simulink model "Trabalho8_2A_Simulink"  (R2022b)
settings: Solver=VariableStepAuto  StartTime=0.0  StopTime=10.0  RelTol=1e-3
undefined symbols (not defined in the file or in its folder): B, C, g, I, L, M, m
settings Model: Creator=brunofavs  LastModifiedBy=brunofavs

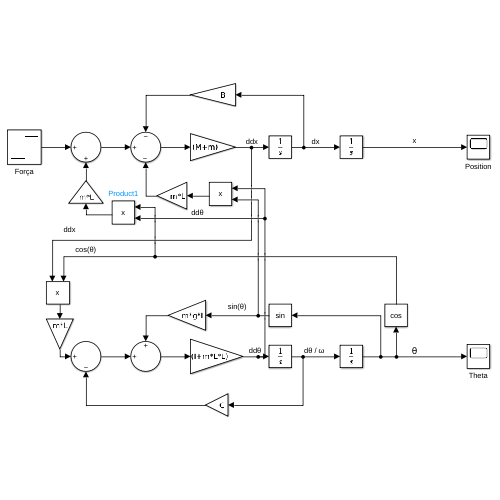
[thumbnail: Simulink's stored preview of the top-level diagram]
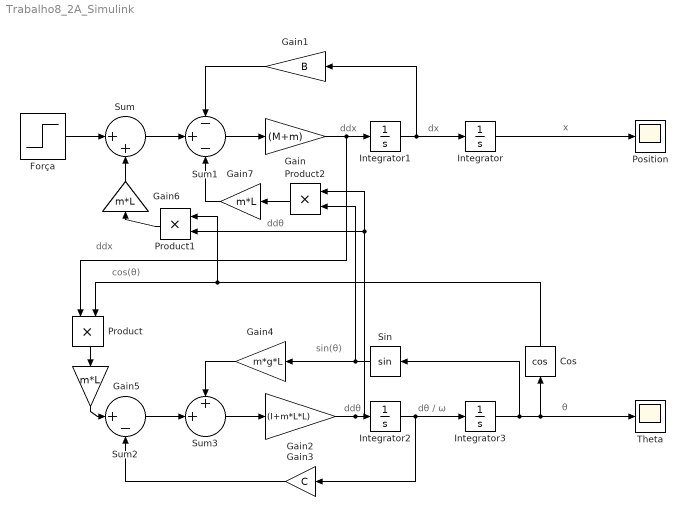
== system Trabalho8_2A_Simulink ==
  note: cos(θ)
  note: sin(θ)
  note: dθ / ω
  note: θ
  note: ddx
  note: dx
  note: x
  note: ddθ
  note: ddx
  note: ddθ
  Cos : Trigonometry  Operator=cos
  Força : Step  After=0.5  SampleTime=0
  Gain : Gain  Gain=(M+m)
  Gain1 : Gain  Gain=B
  Gain2 : Gain  Gain=(I+m*L*L)
  Gain3 : Gain  Gain=C
  Gain4 : Gain  Gain=m*g*L
  Gain5 : Gain  Gain=m*L
  Gain6 : Gain  Gain=m*L
  Gain7 : Gain  Gain=m*L
  Integrator{,1..3} (4 alike) : Integrator
  Position : Scope
  Product : Product
  Product1 : Product
  Product2 : Product
  Sin : Trigonometry
  Sum : Sum  Inputs=|++
  Sum1 : Sum  Inputs=-+-
  Sum2 : Sum  Inputs=|+-
  Sum3 : Sum  Inputs=++|
  Theta : Scope
  wires:
  Integrator1/1 -> Gain1/1, Integrator/1
  Integrator/1 -> Position/1
  Integrator2/1 -> Gain3/1, Integrator3/1
  Integrator3/1 -> Cos/1, Theta/1, Sin/1
  Sum/1 -> Sum1/2
  Força/1 -> Sum/1
  Gain/1 -> Product/1, Integrator1/1
  Sum1/1 -> Gain/1
  Gain1/1 -> Sum1/1
  Gain2/1 -> Product2/1, Product1/2, Integrator2/1
  Sum2/1 -> Sum3/2
  Sum3/1 -> Gain2/1
  Sin/1 -> Product2/2, Gain4/1
  Cos/1 -> Product1/1, Product/2
  Product/1 -> Gain5/1
  Gain5/1 -> Sum2/1
  Gain3/1 -> Sum2/2
  Gain4/1 -> Sum3/1
  Gain6/1 -> Sum/2
  Product1/1 -> Gain6/1
  Gain7/1 -> Sum1/3
  Product2/1 -> Gain7/1
